simulink model "ObjectDetectionBlockMaching"  (R2016a)
settings: Solver=VariableStepAuto  StartTime=0.0  StopTime=10.0  RelTol=1e-3
undefined symbols (not defined in the file): gray, magnitude, none, Rec, SDTV, videoinput
libraries: visionstatistics x2, visionanalysis x1, visionconversions x1, visiontextngfix x1, imaqlib x1
settings Model: Creator=YASARA  LastModifiedBy=YASARA

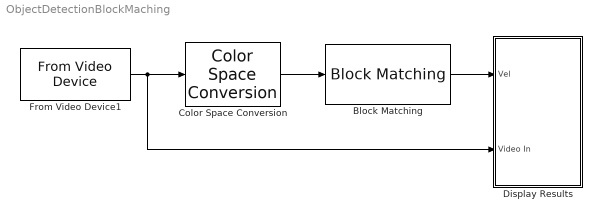
== system ObjectDetectionBlockMaching ==
  Block Matching : visionanalysis/Block Matching  which2img=Current frame and N-th frame back  N=1  searchMethod=Exhaustive  blockSize=[119 159]  overlapping=[0 0]  maxDisplacement=[119 159]  matchCriteria=Mean absolute difference (MAD)  outVelForm=Horizontal and vertical components in complex form  outputMode=Binary point scaling  outputWordLength=8  outputFracLength=0  accumMode=Binary point scaling  accumWordLength=32  accumFracLength=0  prodOutputMode=Binary point scaling  prodOutputWordLength=32  prodOutputFracLength=0  roundingMode=Floor  overflowMode=on
  Color Space Conversion : visionconversions/Color Space  Conversion  conversion=Obsolete  conversionActive=R'G'B' to intensity  wp_str=D65  rec=Rec. 601 (SDTV)  sys=1125/60/2:1  imagePorts=One multidimensional signal
  Display Results : Subsystem
  From Video Device1 : imaqlib/From Video Device  DeviceMenu=winvideo 2 (USB Video Device)  Device=winvideo 2 (USB Video Device)  ObjConstructor=videoinput('winvideo', 2)  VideoFormatMenu=YUY2_160x120  VideoFormat=YUY2_160x120  VideoSource=input1  ROIPosition=[0 0 120 160]  EnableHWTrigger=off  TriggerConfiguration=none/none  SampleTime=1/30  OutputPortsMode=One multidimensional signal  DataType=single  CanDoHWTrigger=no  ReturnedColorSpace=rgb  BlockHandle=154.0001  ROIWidth=160  ROIHeight=120  ROIColumn=0  ROIRow=0  EngXMLPath=C:\Program Files\MATLAB\R2016a\toolbox\imaq\imaq\private  DevXMLPath=C:\MATLAB\SupportPackages\R2016a\toolbox\imaq\supportpackages\genericvideo\adaptor\win64  EngLibPath=C:\Program Files\MATLAB\R2016a\toolbox\imaq\imaqblks\imaqmex\win64  ColorSpace=rgb  BayerSensorAlignment=grbg
  wires:
  Block Matching/1 -> Display Results/1(Vel)
  Color Space Conversion/1 -> Block Matching/1
  From Video Device1/1 -> Display Results/2(Video In), Color Space Conversion/1

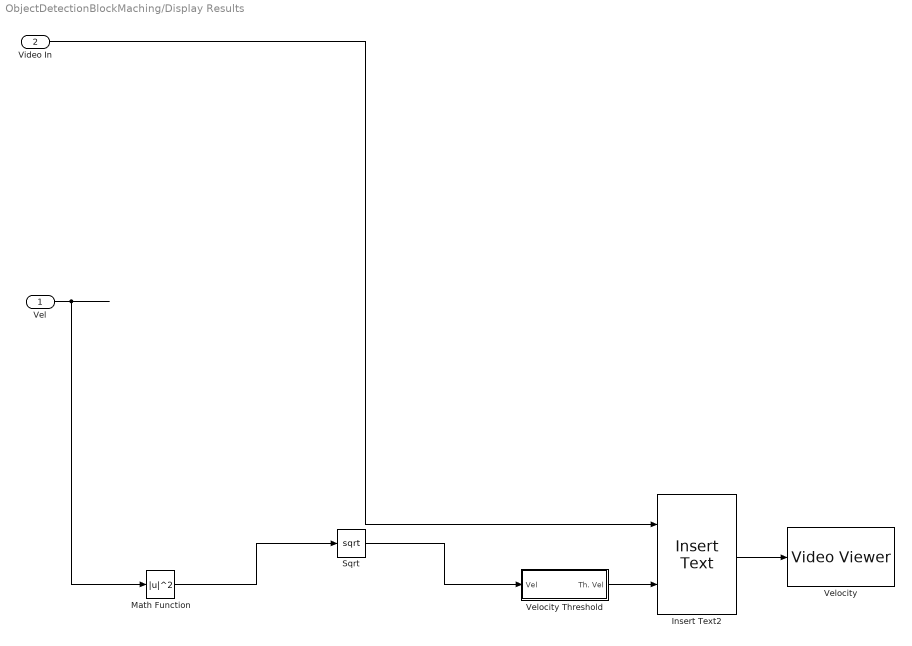
== system ObjectDetectionBlockMaching/Display Results ==
  Vel : Inport
  Video In : Inport  Port=2
  Insert Text2 : visiontextngfix/Insert Text  inputType=Obsolete  theText='velocity : %f'  getTextLocFrom=Specify via dialog  textLoc=[20 10]  getTextColorFrom=Specify via dialog  textColor=[1 1 1]  getTextIntensityFrom=Specify via dialog  textIntensity=1  getTextOpacityFrom=Specify via dialog  textOpacity=1.0  dummyVar2=0  dummyVar3=0  dummyVar4=0  imagePorts=One multidimensional signal  isInputTransposed=off  fontFace=Times New Roman  dummyVar1=0  blockFontSize=16  antiAliased=on
  Math Function : Math  Operator=magnitude^2  SaturateOnIntegerOverflow=on
  Sqrt : Sqrt  SaturateOnIntegerOverflow=on
  Velocity : VideoViewer  colormapValue=gray(256)  FigPos=[68 635 525 420]  trueSizedOnce=on
  Velocity Threshold : Subsystem
  wires:
  Video In/1 -> Insert Text2/1
  Vel/1 -> Math Function/1
  Insert Text2/1 -> Velocity/1
  Velocity Threshold/1(Th. Vel) -> Insert Text2/2
  Math Function/1 -> Sqrt/1
  Sqrt/1 -> Velocity Threshold/1(Vel)

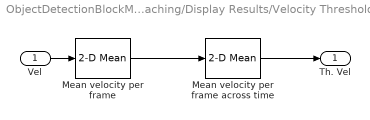
== system ObjectDetectionBlockMaching/Display Results/Velocity Threshold ==
  Vel : Inport
  Mean velocity per frame : visionstatistics/2-D Mean  run=off  reset_popup=None  directionMode=Entire input  dimension=1  treatSBRowAsCol=on  roiEnable=off  roiType=Rectangles  roiPortion=Entire ROI  roiOutput=Individual statistics for each ROI  roiFlag=off  outputDataTypeStr=Inherit: Same as accumulator  outputLastDataTypeStr=Inherit: Same as accumulator  outputMin=[]  outputMax=[]  accumMode=Binary point scaling  accumWordLength=32  accumFracLength=0  accumDataTypeStr=fixdt([],32,0)  accumLastDataTypeStr=fixdt([],32,0)  roundingMode=Floor  overflowMode=off
  Mean velocity per frame across time : visionstatistics/2-D Mean  run=on  reset_popup=None  directionMode=Entire input  dimension=1  treatSBRowAsCol=on  roiEnable=off  roiType=Rectangles  roiPortion=Entire ROI  roiOutput=Individual statistics for each ROI  roiFlag=off  outputDataTypeStr=Inherit: Same as accumulator  outputLastDataTypeStr=Inherit: Same as accumulator  outputMin=[]  outputMax=[]  accumMode=Binary point scaling  accumWordLength=32  accumFracLength=0  accumDataTypeStr=fixdt([],32,0)  accumLastDataTypeStr=fixdt([],32,0)  roundingMode=Floor  overflowMode=off
  Th. Vel : Outport
  wires:
  Mean velocity per frame across time/1 -> Th. Vel/1
  Vel/1 -> Mean velocity per frame/1
  Mean velocity per frame/1 -> Mean velocity per frame across time/1
